simulink model "Subsistema_borroso"  (R2019a)
settings: Solver=ode3  StartTime=0.0  StopTime=10.0  RelTol=1e-3
values from neighbouring files (symbols this model uses):
  Ts = 100e-3    (= 0.1)    [Control_borroso_referencia.m]    (also in Control_borroso_trajectory.m)
libraries: fuzblock x1
settings Model: Creator=mrblissfulgrin  LastModifiedBy=mrblissfulgrin
settings DataIOCC: ReturnWorkspaceOutputs=off

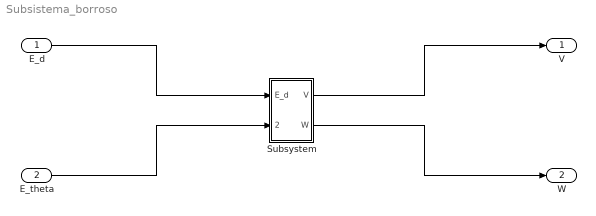
== system Subsistema_borroso ==
  "E_d " : Inport  SampleTime=Ts
  E_theta : Inport  Port=2  SampleTime=Ts
  Subsystem : Subsystem
  "V " : Outport  SampleTime=Ts
  W : Outport  Port=2  SampleTime=Ts
  wires:
  "E_d "/1 -> Subsystem/1("E_d ")
  E_theta/1 -> Subsystem/2(E_theta)
  Subsystem/1("V ") -> "V "/1
  Subsystem/2(W) -> W/1

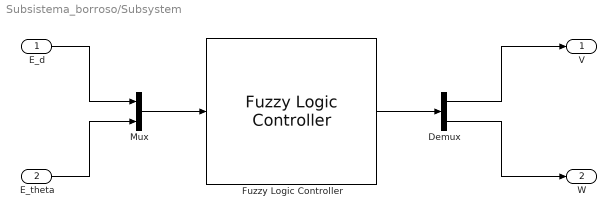
== system Subsistema_borroso/Subsystem ==
  "E_d " : Inport  SampleTime=Ts
  E_theta : Inport  Port=2  SampleTime=Ts
  Demux : Demux  Outputs=2
  Fuzzy Logic Controller : fuzblock/Fuzzy Logic  Controller  FIS='Control_borroso.fis'  OutputSampleNumber=101  DataType=double  FuzzifiedInputs=off  RuleFiringStrengths=off  RuleOutputs=off  AggregatedOutputs=off  SimulateUsing=Interpreted execution  OutOfRangeInputValueMessage=warning  NoRuleFiredMessage=warning  EmptyOutputFuzzySetMessage=warning
  Mux : Mux  Inputs=2
  "V " : Outport  SampleTime=Ts
  W : Outport  Port=2  SampleTime=Ts
  wires:
  Demux/1 -> "V "/1
  Demux/2 -> W/1
  E_theta/1 -> Mux/2
  Mux/1 -> Fuzzy Logic Controller/1
  Fuzzy Logic Controller/1 -> Demux/1
  "E_d "/1 -> Mux/1
